simulink model "class1"  (R2022b)
settings: Solver=VariableStepAuto  StartTime=0.0  StopTime=10.0  RelTol=1e-3
libraries: simulink x1
settings Model: Creator=henry  LastModifiedBy=henry

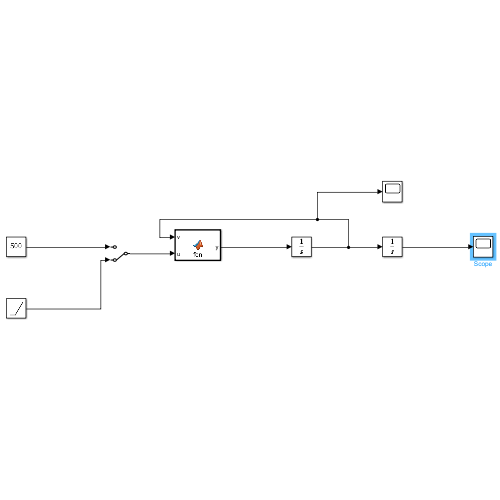
[thumbnail: Simulink's stored preview of the top-level diagram]
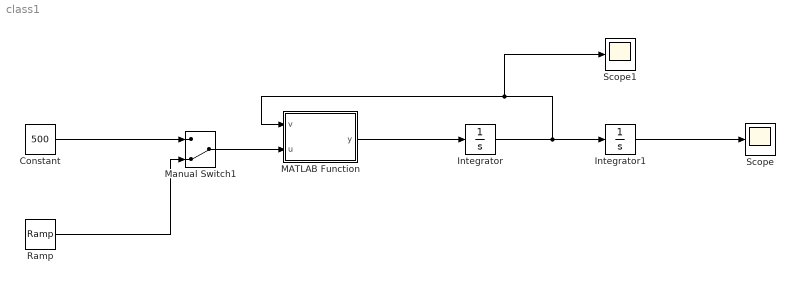
== system class1 ==
  Constant : Constant  Value=500
  Integrator : Integrator  InitialCondition=80*1/3.6
  Integrator1 : Integrator
  MATLAB Function : MATLAB Function  TreatAsAtomicUnit=on
  Manual Switch1 : ManualSwitch  CurrentSetting=0
  Ramp : simulink/Sources/Ramp  slope=1  start=3  InitialOutput=0
  Scope : Scope
  Scope1 : Scope
  wires:
  Integrator1/1 -> Scope/1
  MATLAB Function/1(y) -> Integrator/1
  Integrator/1 -> MATLAB Function/1(v), Scope1/1, Integrator1/1
  Constant/1 -> Manual Switch1/1
  Ramp/1 -> Manual Switch1/2
  Manual Switch1/1 -> MATLAB Function/2(u)

== matlab function class1/MATLAB Function ==
  data: v input; u input; y output
function y = fcn(v, u)
b = 50;
m = 1000;
y = -b/m*v+1/m*u;
